simulink model "Zadatak3_Provjera"  (R2018a)
settings: Solver=VariableStepAuto  StartTime=0.0  StopTime=10.0  RelTol=1e-3
libraries: powerlib x13
settings Model: Creator=Panjevic  LastModifiedBy=Panjevic

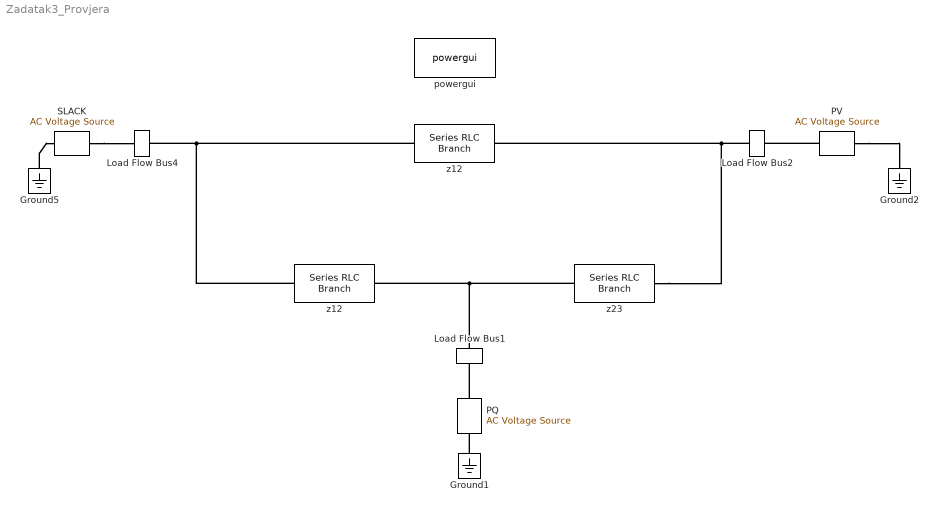
== system Zadatak3_Provjera ==
  Ground1 : powerlib/Elements/Ground  LConnTagsString=a
  Ground2 : powerlib/Elements/Ground  LConnTagsString=a
  Ground5 : powerlib/Elements/Ground  LConnTagsString=a
  Load Flow Bus1 : powerlib/Measurements/Load Flow Bus  LConnTagsString=a  RConnTagsString=a  Phases=A  Connectors=on both sides  ID=BUS_2  Vbase=1  Vref=1  Vangle=0  VLF=1.012  VLFb=NaN  VLFc=NaN  angleLF=-1.584  angleLFb=NaN  angleLFc=NaN
      settings: SourceProductName=Simscape Power Systems
  Load Flow Bus2 : powerlib/Measurements/Load Flow Bus  LConnTagsString=a  RConnTagsString=a  Phases=A  Connectors=on both sides  ID=BUS_3  Vbase=1  Vref=1.03  Vangle=0  VLF=1.03  VLFb=NaN  VLFc=NaN  angleLF=-0.2016  angleLFb=NaN  angleLFc=NaN
      settings: SourceProductName=Simscape Power Systems
  Load Flow Bus4 : powerlib/Measurements/Load Flow Bus  LConnTagsString=a  RConnTagsString=a  Phases=A  Connectors=on both sides  ID=BUS_1  Vbase=1  Vref=1.02  Vangle=0  VLF=1.02  VLFb=NaN  VLFc=NaN  angleLF=0  angleLFb=NaN  angleLFc=NaN
      settings: SourceProductName=Simscape Power Systems
  PQ : powerlib/Electrical Sources/AC Voltage Source  Amplitude=1.01207*1*sqrt(2)  Phase=-1.58412  Frequency=50  SampleTime=0  Measurements=None  BusType=PQ  Pref=-2  Qref=-0.5  Qmin=-inf  Qmax=+inf
  PV : powerlib/Electrical Sources/AC Voltage Source  Amplitude=1.03*1*sqrt(2)  Phase=-0.20158  Frequency=50  SampleTime=0  Measurements=None  BusType=PV  Pref=1.5  Qref=-0.9  Qmin=-inf  Qmax=+inf
  SLACK : powerlib/Electrical Sources/AC Voltage Source  Amplitude=1.02*1*sqrt(2)  Phase=0  Frequency=50  SampleTime=0  Measurements=None  BusType=swing  Pref=-1.4  Qref=-0.9  Qmin=-inf  Qmax=+inf
  powergui : powerlib/powergui  Priority=1  SimulationMode=Phasor  SampleTime=50e-6  frequency=50  Iterations=50  frequencyindice=50  Pbase=100e6  ErrMax=0.0001  UnitsV=kV  UnitsW=MW  buscounter=0  FunctionMessages=off  echomessages=off  EnableUseOfTLC=off  CurrentSourceSwitches=off  DisableSnubberDevices=off  DisableRonSwitches=off  DisableVfSwitches=off  DisplayEquations=off  SolverType=Tustin/Backward Euler (TBE)  Interpol=off  ExternalGateDelay=off  methode=off  Ts=100  x0status=blocks  SPID=on  SwTol=0  HookPort=off  RestoreLinks=warning  ResistiveCurrentMeasurement=off  Frange=[0:2:500]  Ylog=off  Xlog=on  ShowGrid=off  save=off  variable=ZData  structure=0  ZoomFFT=off  StartTime=0.0  cycles=1  DisplayStyle=1  fundamental=60  FreqAxis=off  MaxFrequency=1000  frequencyindicesteady=1  RmsSteady=1  display=off
  z12 : powerlib/Elements/Series RLC Branch  LConnTagsString=__new0  RConnTagsString=__new0  BranchType=RL  Resistance=0.02  Inductance=0.06/(2*pi*50)  SetiL0=off  InitialCurrent=0  Capacitance=0.1  Setx0=off  InitialVoltage=0  Measurements=None
  "z12 " : powerlib/Elements/Series RLC Branch  LConnTagsString=__new0  RConnTagsString=__new0  BranchType=RL  Resistance=0.0059  Inductance=0.0235/(2*pi*50)  SetiL0=off  InitialCurrent=0  Capacitance=0.1  Setx0=off  InitialVoltage=0  Measurements=None
  z23 : powerlib/Elements/Series RLC Branch  LConnTagsString=__new0  RConnTagsString=__new0  BranchType=RL  Resistance=0.0055  Inductance=0.0183/(2*pi*50)  SetiL0=off  InitialCurrent=0  Capacitance=0.1  Setx0=off  InitialVoltage=0  Measurements=None
  connections:
  z12/LConn1 -- Load Flow Bus4/RConn1 -- "z12 "/LConn1
  SLACK/RConn1 -- Load Flow Bus4/LConn1
  Ground5/LConn1 -- SLACK/LConn1
  Ground1/LConn1 -- PQ/LConn1
  PQ/RConn1 -- Load Flow Bus1/RConn1
  Load Flow Bus1/LConn1 -- z12/RConn1 -- z23/LConn1
  Load Flow Bus2/LConn1 -- z23/RConn1 -- "z12 "/RConn1
  PV/RConn1 -- Load Flow Bus2/RConn1
  PV/LConn1 -- Ground2/LConn1
